simulink model "Adaptive_Final"  (R2025b)
settings: Solver=VariableStepAuto  StartTime=0.0  StopTime=10.0  RelTol=1e-3
values from neighbouring files (symbols this model uses):
  bitDelay = symbolDelay * k    [Adaptive.m]    (also in adaptive.m; runsim.m)
undefined symbols (not defined in the file or in its folder): doppler, QAM
libraries: commchan3 x2, commdigbbndam3 x2, commfilt2 x2, commsink2 x1, simulink x1, commrandsrc3 x1
settings Model: Creator=namit  LastModifiedBy=namit

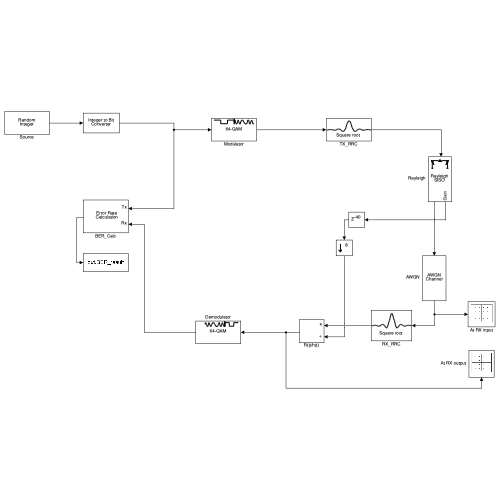
[thumbnail: Simulink's stored preview of the top-level diagram]
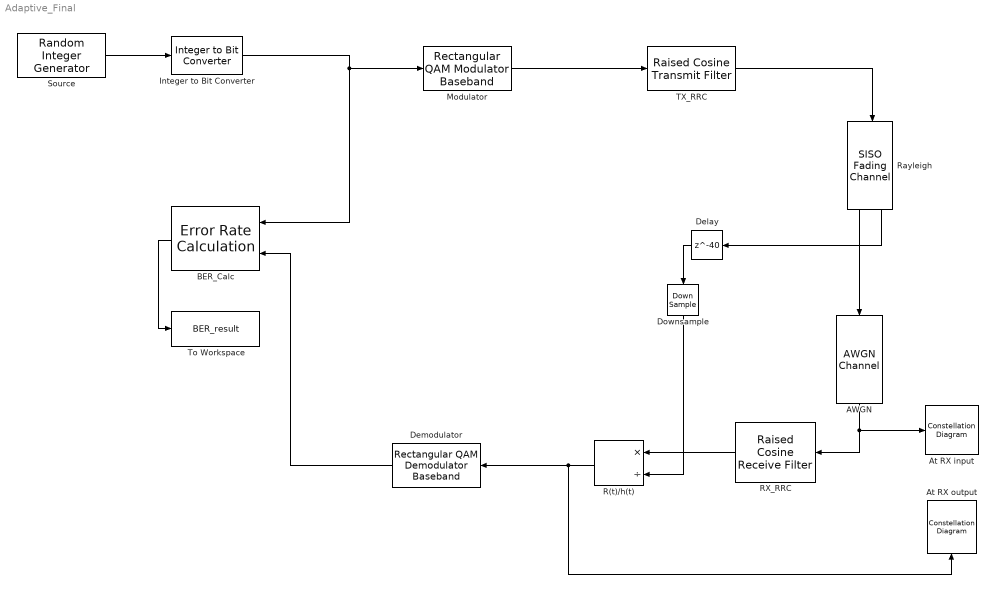
== system Adaptive_Final ==
  AWGN : commchan3/AWGN Channel  LegacyMode=off  NoiseMethod="Signal to noise ratio  (SNR)"  noiseMode="Signal to noise ratio  (SNR)"  EbNo=36  EsNo=10  SNR=current_snr  BitsPerSymbol=1  SignalPower=1  SpecifySymbolPeriod=off  SamplesPerSymbol=1  SymbolPeriod=1  VarianceSource=Input port  Variance=1  RandomStream=Global stream  Seed=67  SimulateUsing=Interpreted execution
  At RX input : ConstellationDiagram  WindowPosition=[756.000000,82.000000,707.000000,809.000000,]  Visible=on  ScopeFrameLocation=window  ReferenceConstellation=64-QAM  XLimits=[-1.375,1.375]  YLimits=[-1.375,1.375]  AxesLimits=[-1.375,1.375]  MaximizeAxes=on
  At RX output : ConstellationDiagram  WindowPosition=[28.000000,89.000000,727.000000,798.000000,]  Visible=on  ScopeFrameLocation=window  ReferenceConstellation=64-QAM  XLimits=[-1.5026448932837324,1.4711099473198885]  YLimits=[-1.5026448932837324,1.4711099473198885]  AxesLimits=[-1.5026448932837324,1.4711099473198885]  MaximizeAxes=on
  BER_Calc : commsink2/Error Rate Calculation  N=bitDelay  st_delay=60  cp_mode=Entire frame  subframe=[]  PMode=Port  WsName=ErrorVec  RsMode2=off  stop=on  numErr=100  maxBits=1e6
  Delay : Delay  DelayLength=40  InputProcessing=Columns as channels (frame based)
  Demodulator : commdigbbndam3/Rectangular QAM Demodulator Baseband  M=64  OutType=Bit  DecType=Hard decision  VarSource=Dialog  Variance=1  Dec=Gray  Mapping=[0:15]  PowType=Average Power  MinDist=2  AvgPow=1  PeakPow=1  Ph=0  outDtype1=Inherit via internal rule  outDtype2=Inherit via internal rule  derotateFactorWordLen=16  derotateFactorDataTypeStr=Inherit: Same word length as input  derotateFactorLastDataTypeStr=Inherit: Same word length as input  denormFactorWordLen=16  denormFactorDataTypeStr=Inherit: Same word length as input  denormFactorLastDataTypeStr=Inherit: Same word length as input  prodOutWordLen=32  prodOutOverflowMode=Wrap  prodOutRoundingMode=Floor  prodOutOvFlMode=off  prodOutOvFlModeLastStrValue=off  sumWordLen=32
  Downsample : DownSample  N=8
  Integer to Bit Converter : simulink/Logic and Bit Operations/Integer to Bit Converter  nbits=6  signedInputValues=Unsigned  bitOrder=MSB first  outDtype=Inherit via internal rule
  Modulator : commdigbbndam3/Rectangular QAM Modulator Baseband  M=64  InType=Bit  Enc=Gray  Mapping=[0:15]  PowType=Average Power  MinDist=2  AvgPow=1  PeakPow=1  Ph=0  outDtype=double  outWordLen=16  outUDDataType=sfix(16)  outFracLenMode=Best precision  outFracLen=15  outDataTypeStr=double  outLastDataTypeStr=double
  R(t)/h(t) : Product  Inputs=*/
  RX_RRC : commfilt2/Raised Cosine Receive Filter  filtType=Square root  R=0.2  filtSpan=10  N=8  downFactor=8  downOffset=0  filterGain=1  InputProcessing=Columns as channels (frame based)  RateOptions=Enforce single-rate processing  framing=Mute  checkCoeff=off  variableName=rcRxFilt  currentFiltSpan=10  D=5  inputOffset=0  sampMode=Mute  saveAsFlag=0  rateMode=Downsampling  checkGain=Normalized  launchFVT=on  roundingMode=Floor  overflowMode=off  coeffDataTypeStr=Inherit: Same word length as input  coeffMin=[]  coeffMax=[]  coeffLastDataTypeStr=Inherit: Same word length as input  accumDataTypeStr=Inherit: Same as product output  accumLastDataTypeStr=Inherit: Same as product output  outputDataTypeStr=Inherit: Same as accumulator  outputMin=[]  outputMax=[]  outputLastDataTypeStr=Inherit: Same as accumulator
  Rayleigh : commchan3/SISO Fading Channel  InheritSampleRate=on  SampleRate=1  PathDelays=0  AveragePathGains=0  NormalizePathGains=on  FadingDistribution=Rayleigh  KFactor=3  DirectPathDopplerShift=0  DirectPathInitialPhase=0  MaximumDopplerShift=0.05  DopplerSpectrum=doppler('Jakes')  RandomStream=mt19937ar with seed  Seed=73  PathGainsOutputPort=on  ChannelFilterDelayOutputPort=off  SimulateUsing=Interpreted execution  Visualization=Off  PathsForDopplerDisplay=1  SamplesToDisplay=25%
  Source : commrandsrc3/Random Integer Generator  SetSize=64  SeedSource=Auto  Seed=0  SampleTime=1  SamplesPerFrame=1998  OutputDataType=double  SimulateUsing=Interpreted execution
  TX_RRC : commfilt2/Raised Cosine Transmit Filter  filtType=Square root  R=0.2  filtSpan=10  N=8  filterGain=1  InputProcessing=Columns as channels (frame based)  RateOptions=Enforce single-rate processing  framing=Mute  checkCoeff=off  variableName=rcTxFilt  checkGain=Normalized  sampMode=Mute  saveAsFlag=0  currentFiltSpan=10  D=(10)/2  launchFVT=on  roundingMode=Floor  overflowMode=off  coeffDataTypeStr=Inherit: Same word length as input  coeffMin=[]  coeffMax=[]  coeffLastDataTypeStr=Inherit: Same word length as input  outputDataTypeStr=Inherit: Same as accumulator  outputMin=[]  outputMax=[]  outputLastDataTypeStr=Inherit: Same as accumulator
  To Workspace : ToWorkspace  VariableName=BER_result  SampleTime=-1
      settings: MaxDataPoints=1
  wires:
  Modulator/1 -> TX_RRC/1
  AWGN/1 -> At RX input/1, RX_RRC/1
  Source/1 -> Integer to Bit Converter/1
  Integer to Bit Converter/1 -> BER_Calc/1, Modulator/1
  BER_Calc/1 -> To Workspace/1
  TX_RRC/1 -> Rayleigh/1
  Rayleigh/1 -> AWGN/1
  R(t)/h(t)/1 -> At RX output/1, Demodulator/1
  RX_RRC/1 -> R(t)/h(t)/1
  Rayleigh/2 -> Delay/1
  Delay/1 -> Downsample/1
  Downsample/1 -> R(t)/h(t)/2
  Demodulator/1 -> BER_Calc/2
